simulink model "master_thesis_simulink"  (R2022a)
settings: Solver=VariableStepAuto  StartTime=0.0  StopTime=p_0p.time(end)  FixedStep=0.001  RelTol=1e-3
values from neighbouring files (symbols this model uses):
  markers_forearm = [0.00210510253906 -0.143263397217 -0.00798474121094]    [markers_forearm.mat]
  markers_shoulder = [0.010127746582 -0.151647644043 -0.0119686279297]    [markers_shoulder.mat]
undefined symbols (not defined in the file or in its folder): arm, DiscIntNeverNeededParam, Discrete, ekf, kf, LS, m, markers_hand, n, noise, q0, q0_LS, q0_model, sample_Time, selected, state_observer, Time, tSh_0_0Conf, X, Y, Z
libraries: sm_lib x2029, nesl_utility x1553, robotlib x75, ctrlSharedLib x8
(part 1 of 70)
settings Model: Creator=gioel  LastModifiedBy=gioel
settings DebuggingCC: SignalInfNanChecking=error  InheritedTsInSrcMsg=none

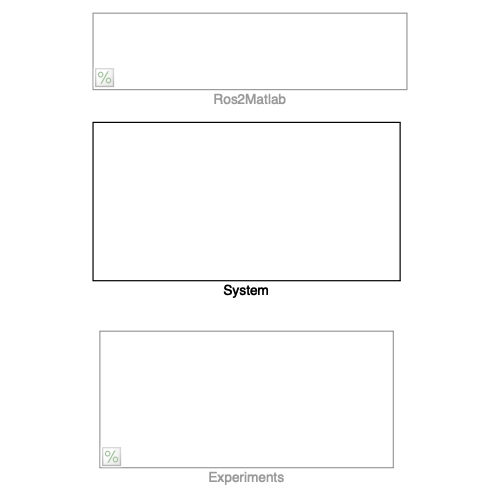
[thumbnail: Simulink's stored preview of the top-level diagram]
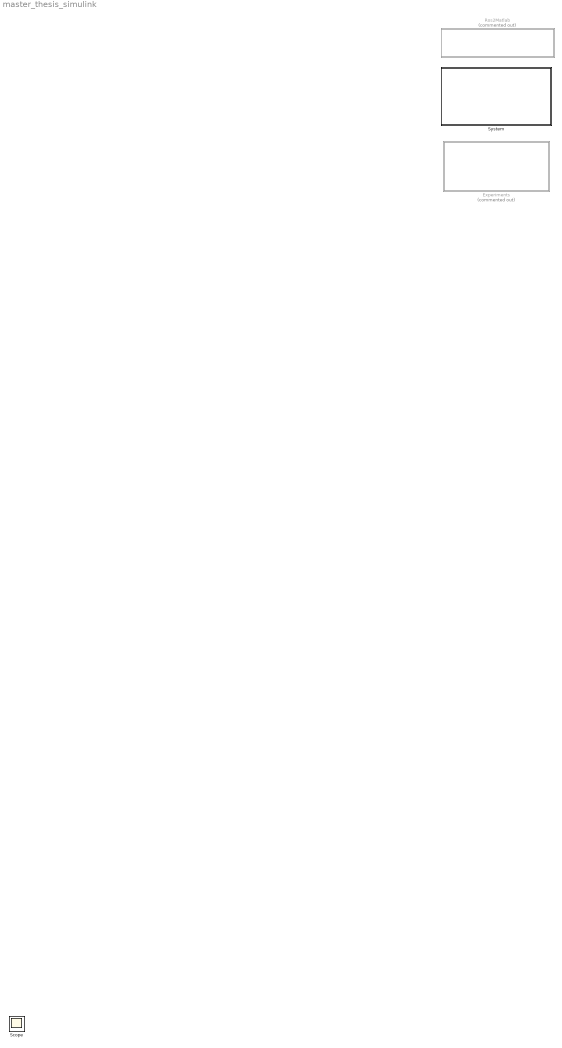
== system master_thesis_simulink ==
  Experiments : Subsystem  Commented=on
  Ros2Matlab : Subsystem  Commented=on
  System : Subsystem
  Scope : Scope

== system master_thesis_simulink/Experiments ==
  S0_F1_H2 : Subsystem  Commented=on
  S0_F2_H2 : Subsystem  Commented=on
  S1_F0_H2 : Subsystem  Commented=on
  S1_F0_H3 : Subsystem  Commented=on
  S1_F1_H2 : Subsystem
  S1_F2_H2 : Subsystem  Commented=on
  S2_F0_H2 : Subsystem  Commented=on

== system master_thesis_simulink/Ros2Matlab ==
  S0_F1_H2 : Subsystem  Commented=on
  S0_F2_H2 : Subsystem  Commented=on
  S1_F0_H2 : Subsystem  Commented=on
  S1_F0_H3 : Subsystem  Commented=on
  S1_F1_H2 : Subsystem
  S1_F2_H2 : Subsystem  Commented=on
  S2_F0_H2 : Subsystem  Commented=on

== system master_thesis_simulink/System ==
  note: q1 = shoulder_x
      | q2 = shoulder_y
      | q3 = shoulder_z
      | q4 = elbow_x
      | q5 = wrist_x
      | q6 = wrist_y
      | q7 = wrist_z
  Constant1 : Constant  Value=markers_shoulder
  Constant2 : Constant  Value=markers_forearm
  Constant3 : Constant  Value=markers_hand
  EKF : Subsystem  Commented=on
  EKF1 : Subsystem  Commented=on
  Human arm : Subsystem  Commented=on
  LKF : Subsystem  Commented=on
  LS : Subsystem  Commented=on
  Mux1 : Mux  Inputs=7
  Mux4 : Mux  Inputs=7
  Noisy p : Subsystem  Commented=on
  Noisy pdot : Subsystem  Commented=on
  Ref : FromWorkspace  Commented=on  VariableName=q_trajectory
  Scope : Scope  NumInputPorts=2
  Scope1 : Scope  NumInputPorts=4
  Show Results : Subsystem
  To Workspace : ToWorkspace  VariableName=q  SaveFormat=Structure With Time  SampleTime=-1
  To Workspace2 : ToWorkspace  VariableName=p  SaveFormat=Structure With Time  SampleTime=-1
  To Workspace4 : ToWorkspace  VariableName=qdot  SaveFormat=Structure With Time  SampleTime=-1
  To Workspace6 : ToWorkspace  VariableName=pdot  SaveFormat=Structure With Time  SampleTime=-1
  ZOH : ZeroOrderHold  SampleTime=sample_Time
  ZOH1 : ZeroOrderHold  SampleTime=sample_Time
  ZOH_q : ZeroOrderHold  SampleTime=sample_Time
  tag scope: markers_f=global, markers_h=global, markers_s=global, p=global, p_true=global, pdot=global, pdot_true=global, q=global, qdot=global
  wires:
  Constant1/1 -> [markers_s]
  [qdot6] -> Mux4/6
  [qdot5] -> Mux4/5
  Constant3/1 -> [markers_h]
  [q6] -> Mux1/6
  Constant2/1 -> [markers_f]
  [qdot2] -> Mux4/2
  [q4] -> Mux1/4
  [q7] -> Mux1/7
  Mux4/1 -> [qdot], To Workspace4/1
  [q2] -> Mux1/2
  [q3] -> Mux1/3
  [q1] -> Mux1/1
  [qdot1] -> Mux4/1
  [q5] -> Mux1/5
  [qdot3] -> Mux4/3
  [qdot7] -> Mux4/7
  [qdot4] -> Mux4/4
  [q] -> Scope1/1  "q"
  ZOH/1 -> EKF1/1(u_noisyk), EKF/1(pdot_k), LKF/1(pdot_k)  "pdot_k"
  Human arm/1(p) -> Scope/1, Noisy p/1(p_true), [p_true]  "p_true"
  Human arm/2(pdot) -> Noisy pdot/1(pdot_true), [pdot_true]  "pdot_true"
  LS/1(q_LS) -> Scope1/2  "q_LS"
  EKF/1(" ") -> Scope1/4  "q_EKF"
  [p] -> ZOH1/1
  ZOH1/1 -> EKF1/2(p_noisyk), EKF/2(p_k), LKF/2(p_k)  "p_k"
  [pdot] -> LS/1(pdot), ZOH/1
  Noisy p/1(p) -> Scope/2, [p], To Workspace2/1  "p"
  Noisy pdot/1(pdot) -> To Workspace6/1, [pdot]  "pdot"
  Ref/1 -> Human arm/1(q ref)
  LKF/1(q_KF) -> Scope1/3
  Mux1/1 -> ZOH_q/1
  ZOH_q/1 -> [q], To Workspace/1  "q_k"

== system master_thesis_simulink/Experiments/S0_F1_H2 ==
  Constant : Constant  Value=selected
  Experiments : Subsystem  TreatAsAtomicUnit=on
  If1 : If
  If2 : If
  If3 : If
  MATLAB Function3 : MATLAB Function  TreatAsAtomicUnit=on
  Model validation : Subsystem  Commented=on  TreatAsAtomicUnit=on
  Noise estimation : Subsystem  Commented=on  TreatAsAtomicUnit=on
  Reshape{1,3..5,7..10} (8 alike) : Reshape  OutputDimensionality=Customize  OutputDimensions=[6,6]
  Scope : Scope
  Selector{,2..4,6..9} (8 alike) : Selector  NumberOfDimensions=2  InputPortWidth=36  IndexOptions=Index vector (dialog),Index vector (dialog)  Indices=1:3,1:3  OutputSizes=1,1
  Terminator1 : Terminator
  Terminator2 : Terminator
  Terminator3 : Terminator
  Vector Concatenate1 : Concatenate  NumInputs=3  Mode=Multidimensional array
  Vector Concatenate2 : Concatenate  NumInputs=3  Mode=Multidimensional array
  tag scope: Rpi_W=global, Rvi_W=global
  wires:
  Selector4/1 -> Vector Concatenate1/3
  Reshape5/1 -> Selector4/1
  Vector Concatenate1/1 -> [Rpi_W]
  Constant/1 -> Experiments/3(Selector)
  If2/1 -> Model validation/Action
  If1/1 -> Experiments/Action
  If3/2 -> Terminator2/1
  Selector3/1 -> Vector Concatenate1/2
  Reshape4/1 -> Selector3/1
  [Rpi_W] -> Noise estimation/2(Rpi_W)
  [isNew] -> MATLAB Function3/1(isNew)
  [Rp3_W] -> Reshape4/1
  If3/1 -> Noise estimation/Action
  Selector/1 -> Noise estimation/1(Rp0_W)
  Reshape1/1 -> Selector/1
  Reshape3/1 -> Selector2/1
  MATLAB Function3/1(y) -> If3/1, If2/1, Scope/1, If1/1
  [v_0p] -> Experiments/2(v_0')
  [Rp0_W] -> Reshape1/1
  If2/2 -> Terminator1/1
  [Rp4_W] -> Reshape5/1
  [Rp2_W] -> Reshape3/1
  If1/2 -> Terminator3/1
  Selector2/1 -> Vector Concatenate1/1
  Selector6/1 -> Vector Concatenate2/1
  [Rv2_W] -> Reshape7/1
  [Rv4_W] -> Reshape9/1
  Reshape7/1 -> Selector6/1
  [Rv3_W] -> Reshape8/1
  Reshape8/1 -> Selector7/1
  Selector7/1 -> Vector Concatenate2/2
  Vector Concatenate2/1 -> [Rvi_W]
  Reshape9/1 -> Selector8/1
  Selector8/1 -> Vector Concatenate2/3
  [Rvi_W] -> Noise estimation/4(Rvi_W)
  [Rv0_W] -> Reshape10/1
  Reshape10/1 -> Selector9/1
  Selector9/1 -> Noise estimation/3(Rv0_W)
  [p_0p] -> Model validation/1(p_0'), Experiments/1(p_0')

== system master_thesis_simulink/Experiments/S0_F2_H2 ==
  Constant : Constant  Value=selected
  Experiments : Subsystem  Commented=on  TreatAsAtomicUnit=on
  If1 : If
  If2 : If
  If3 : If
  MATLAB Function3 : MATLAB Function  TreatAsAtomicUnit=on
  Model validation : Subsystem  TreatAsAtomicUnit=on
  Noise estimation : Subsystem  Commented=on  TreatAsAtomicUnit=on
  Reshape{1..10} (10 alike) : Reshape  OutputDimensionality=Customize  OutputDimensions=[6,6]
  Scope : Scope
  Selector{,1..9} (10 alike) : Selector  NumberOfDimensions=2  InputPortWidth=36  IndexOptions=Index vector (dialog),Index vector (dialog)  Indices=1:3,1:3  OutputSizes=1,1
  Terminator1 : Terminator
  Terminator2 : Terminator
  Terminator3 : Terminator
  Vector Concatenate1 : Concatenate  NumInputs=4  Mode=Multidimensional array
  Vector Concatenate2 : Concatenate  NumInputs=4  Mode=Multidimensional array
  tag scope: Rpi_W=global, Rvi_W=global
  wires:
  [p_0p] -> Experiments/1(p_0'), Model validation/1(p_0')
  Selector9/1 -> Noise estimation/3(Rv0_W)
  Reshape10/1 -> Selector9/1
  [Rv0_W] -> Reshape10/1
  [Rvi_W] -> Noise estimation/4(Rvi_W)
  Selector8/1 -> Vector Concatenate2/4
  Reshape9/1 -> Selector8/1
  Vector Concatenate2/1 -> [Rvi_W]
  [Rv1_W] -> Reshape6/1
  Selector7/1 -> Vector Concatenate2/3
  Reshape8/1 -> Selector7/1
  [Rv3_W] -> Reshape8/1
  Reshape7/1 -> Selector6/1
  Reshape6/1 -> Selector5/1
  [Rv4_W] -> Reshape9/1
  Selector5/1 -> Vector Concatenate2/1
  [Rv2_W] -> Reshape7/1
  Selector6/1 -> Vector Concatenate2/2
  Selector2/1 -> Vector Concatenate1/2
  If1/2 -> Terminator3/1
  [Rp2_W] -> Reshape3/1
  Selector1/1 -> Vector Concatenate1/1
  [Rp4_W] -> Reshape5/1
  If2/2 -> Terminator1/1
  Reshape2/1 -> Selector1/1
  [Rp0_W] -> Reshape1/1
  [v_0p] -> Experiments/2(v_0')
  MATLAB Function3/1(y) -> If1/1, Scope/1, If2/1, If3/1
  Reshape3/1 -> Selector2/1
  Reshape1/1 -> Selector/1
  Selector/1 -> Noise estimation/1(Rp0_W)
  If3/1 -> Noise estimation/Action
  [Rp3_W] -> Reshape4/1
  [isNew] -> MATLAB Function3/1(isNew)
  [Rpi_W] -> Noise estimation/2(Rpi_W)
  Reshape4/1 -> Selector3/1
  Selector3/1 -> Vector Concatenate1/3
  If3/2 -> Terminator2/1
  [Rp1_W] -> Reshape2/1
  If1/1 -> Experiments/Action
  If2/1 -> Model validation/Action
  Constant/1 -> Experiments/3(Selector)
  Vector Concatenate1/1 -> [Rpi_W]
  Reshape5/1 -> Selector4/1
  Selector4/1 -> Vector Concatenate1/4

== system master_thesis_simulink/Experiments/S1_F0_H2 ==
  Constant : Constant  Value=selected
  Experiments : Subsystem  TreatAsAtomicUnit=on
  If1 : If
  If2 : If
  If3 : If
  MATLAB Function3 : MATLAB Function  TreatAsAtomicUnit=on
  Model validation : Subsystem  Commented=on  TreatAsAtomicUnit=on
  Noise estimation : Subsystem  Commented=on  TreatAsAtomicUnit=on
  Reshape{1..2,4..6,8..10} (8 alike) : Reshape  OutputDimensionality=Customize  OutputDimensions=[6,6]
  Scope : Scope
  Selector{,1,3..5,7..9} (8 alike) : Selector  NumberOfDimensions=2  InputPortWidth=36  IndexOptions=Index vector (dialog),Index vector (dialog)  Indices=1:3,1:3  OutputSizes=1,1
  Terminator1 : Terminator
  Terminator2 : Terminator
  Terminator3 : Terminator
  Vector Concatenate1 : Concatenate  NumInputs=3  Mode=Multidimensional array
  Vector Concatenate2 : Concatenate  NumInputs=3  Mode=Multidimensional array
  tag scope: Rpi_W=global, Rvi_W=global
  wires:
  Selector4/1 -> Vector Concatenate1/3
  Reshape5/1 -> Selector4/1
  Vector Concatenate1/1 -> [Rpi_W]
  Constant/1 -> Experiments/3(Selector)
  If2/1 -> Model validation/Action
  If1/1 -> Experiments/Action
  [Rp1_W] -> Reshape2/1
  If3/2 -> Terminator2/1
  Selector3/1 -> Vector Concatenate1/2
  Reshape4/1 -> Selector3/1
  [Rpi_W] -> Noise estimation/2(Rpi_W)
  [isNew] -> MATLAB Function3/1(isNew)
  [Rp3_W] -> Reshape4/1
  If3/1 -> Noise estimation/Action
  Selector/1 -> Noise estimation/1(Rp0_W)
  Reshape1/1 -> Selector/1
  MATLAB Function3/1(y) -> If3/1, If2/1, Scope/1, If1/1
  [v_0p] -> Experiments/2(v_0')
  [Rp0_W] -> Reshape1/1
  Reshape2/1 -> Selector1/1
  If2/2 -> Terminator1/1
  [Rp4_W] -> Reshape5/1
  Selector1/1 -> Vector Concatenate1/1
  If1/2 -> Terminator3/1
  Selector5/1 -> Vector Concatenate2/1
  [Rv4_W] -> Reshape9/1
  Reshape6/1 -> Selector5/1
  [Rv3_W] -> Reshape8/1
  Reshape8/1 -> Selector7/1
  Selector7/1 -> Vector Concatenate2/2
  [Rv1_W] -> Reshape6/1
  Vector Concatenate2/1 -> [Rvi_W]
  Reshape9/1 -> Selector8/1
  Selector8/1 -> Vector Concatenate2/3
  [Rvi_W] -> Noise estimation/4(Rvi_W)
  [Rv0_W] -> Reshape10/1
  Reshape10/1 -> Selector9/1
  Selector9/1 -> Noise estimation/3(Rv0_W)
  [p_0p] -> Model validation/1(p_0'), Experiments/1(p_0')

== system master_thesis_simulink/Experiments/S1_F0_H3 ==
  Constant : Constant  Value=selected
  Experiments : Subsystem  Commented=on  TreatAsAtomicUnit=on
  If1 : If
  If2 : If
  If3 : If
  MATLAB Function3 : MATLAB Function  TreatAsAtomicUnit=on
  Model validation : Subsystem  Commented=on  TreatAsAtomicUnit=on
  Noise estimation : Subsystem  TreatAsAtomicUnit=on
  Reshape{1..10} (10 alike) : Reshape  OutputDimensionality=Customize  OutputDimensions=[6,6]
  Scope : Scope
  Selector{,1..9} (10 alike) : Selector  NumberOfDimensions=2  InputPortWidth=36  IndexOptions=Index vector (dialog),Index vector (dialog)  Indices=1:3,1:3  OutputSizes=1,1
  Terminator1 : Terminator
  Terminator2 : Terminator
  Terminator3 : Terminator
  Vector Concatenate1 : Concatenate  NumInputs=4  Mode=Multidimensional array
  Vector Concatenate2 : Concatenate  NumInputs=4  Mode=Multidimensional array
  tag scope: Rpi_W=global, Rvi_W=global
  wires:
  Selector4/1 -> Vector Concatenate1/4
  Reshape5/1 -> Selector4/1
  Vector Concatenate1/1 -> [Rpi_W]
  Constant/1 -> Experiments/3(Selector)
  If2/1 -> Model validation/Action
  If1/1 -> Experiments/Action
  [Rp1_W] -> Reshape2/1
  If3/2 -> Terminator2/1
  Selector3/1 -> Vector Concatenate1/3
  Reshape4/1 -> Selector3/1
  [Rpi_W] -> Noise estimation/2(Rpi_W)
  [isNew] -> MATLAB Function3/1(isNew)
  [Rp3_W] -> Reshape4/1
  If3/1 -> Noise estimation/Action
  Selector/1 -> Noise estimation/1(Rp0_W)
  Reshape1/1 -> Selector/1
  Reshape3/1 -> Selector2/1
  MATLAB Function3/1(y) -> If3/1, If2/1, Scope/1, If1/1
  [v_0p] -> Experiments/2(v_0')
  [Rp0_W] -> Reshape1/1
  Reshape2/1 -> Selector1/1
  If2/2 -> Terminator1/1
  [Rp4_W] -> Reshape5/1
  Selector1/1 -> Vector Concatenate1/1
  [Rp2_W] -> Reshape3/1
  If1/2 -> Terminator3/1
  Selector2/1 -> Vector Concatenate1/2
  Selector6/1 -> Vector Concatenate2/2
  [Rv2_W] -> Reshape7/1
  Selector5/1 -> Vector Concatenate2/1
  [Rv4_W] -> Reshape9/1
  Reshape6/1 -> Selector5/1
  Reshape7/1 -> Selector6/1
  [Rv3_W] -> Reshape8/1
  Reshape8/1 -> Selector7/1
  Selector7/1 -> Vector Concatenate2/3
  [Rv1_W] -> Reshape6/1
  Vector Concatenate2/1 -> [Rvi_W]
  Reshape9/1 -> Selector8/1
  Selector8/1 -> Vector Concatenate2/4
  [Rvi_W] -> Noise estimation/4(Rvi_W)
  [Rv0_W] -> Reshape10/1
  Reshape10/1 -> Selector9/1
  Selector9/1 -> Noise estimation/3(Rv0_W)
  [p_0p] -> Model validation/1(p_0'), Experiments/1(p_0')

== system master_thesis_simulink/Experiments/S1_F1_H2 ==
  Constant : Constant  Value=selected
  Experiments : Subsystem  TreatAsAtomicUnit=on
  Human arm1 : Subsystem
  If1 : If
  If2 : If
  If3 : If
  MATLAB Function3 : MATLAB Function  TreatAsAtomicUnit=on
  Model validation : Subsystem  Commented=on  TreatAsAtomicUnit=on
  Noise estimation : Subsystem  Commented=on  TreatAsAtomicUnit=on
  Reshape{1..10} (10 alike) : Reshape  OutputDimensionality=Customize  OutputDimensions=[6,6]
  Scope : Scope
  Selector{,1..9} (10 alike) : Selector  NumberOfDimensions=2  InputPortWidth=36  IndexOptions=Index vector (dialog),Index vector (dialog)  Indices=1:3,1:3  OutputSizes=1,1
  Terminator1 : Terminator
  Terminator2 : Terminator
  Terminator3 : Terminator
  Vector Concatenate1 : Concatenate  NumInputs=4  Mode=Multidimensional array
  Vector Concatenate2 : Concatenate  NumInputs=4  Mode=Multidimensional array
  tag scope: Rpi_W=global, Rvi_W=global
  wires:
  Selector4/1 -> Vector Concatenate1/4
  Reshape5/1 -> Selector4/1
  Vector Concatenate1/1 -> [Rpi_W]
  Constant/1 -> Experiments/3(Selector)
  If2/1 -> Model validation/Action
  If1/1 -> Experiments/Action
  [Rp1_W] -> Reshape2/1
  If3/2 -> Terminator2/1
  Selector3/1 -> Vector Concatenate1/3
  Reshape4/1 -> Selector3/1
  [Rpi_W] -> Noise estimation/2(Rpi_W)
  [isNew] -> MATLAB Function3/1(isNew)
  [Rp3_W] -> Reshape4/1
  If3/1 -> Noise estimation/Action
  Selector/1 -> Noise estimation/1(Rp0_W)
  Reshape1/1 -> Selector/1
  Reshape3/1 -> Selector2/1
  MATLAB Function3/1(y) -> If3/1, If2/1, Scope/1, If1/1
  [v_0p] -> Experiments/2(v_0')
  [Rp0_W] -> Reshape1/1
  Reshape2/1 -> Selector1/1
  If2/2 -> Terminator1/1
  [Rp4_W] -> Reshape5/1
  Selector1/1 -> Vector Concatenate1/1
  [Rp2_W] -> Reshape3/1
  If1/2 -> Terminator3/1
  Selector2/1 -> Vector Concatenate1/2
  Selector6/1 -> Vector Concatenate2/2
  [Rv2_W] -> Reshape7/1
  Selector5/1 -> Vector Concatenate2/1
  [Rv4_W] -> Reshape9/1
  Reshape6/1 -> Selector5/1
  Reshape7/1 -> Selector6/1
  [Rv3_W] -> Reshape8/1
  Reshape8/1 -> Selector7/1
  Selector7/1 -> Vector Concatenate2/3
  [Rv1_W] -> Reshape6/1
  Vector Concatenate2/1 -> [Rvi_W]
  Reshape9/1 -> Selector8/1
  Selector8/1 -> Vector Concatenate2/4
  [Rvi_W] -> Noise estimation/4(Rvi_W)
  [Rv0_W] -> Reshape10/1
  Reshape10/1 -> Selector9/1
  Selector9/1 -> Noise estimation/3(Rv0_W)
  [p_0p] -> Model validation/1(p_0'), Experiments/1(p_0')
  Experiments/1(Output) -> Human arm1/1(q_EKF)

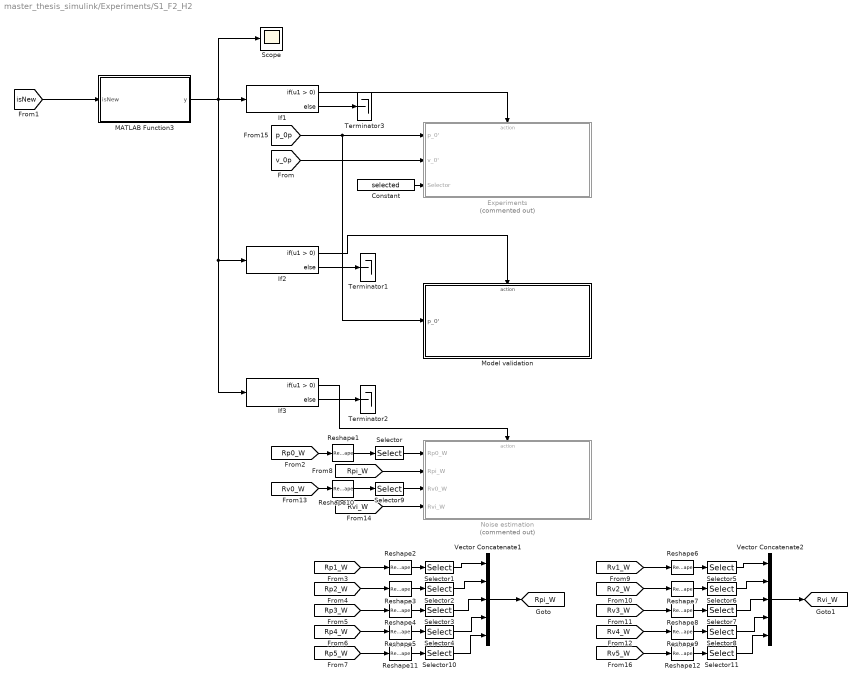
== system master_thesis_simulink/Experiments/S1_F2_H2 ==
  Constant : Constant  Value=selected
  Experiments : Subsystem  Commented=on  TreatAsAtomicUnit=on
  If1 : If
  If2 : If
  If3 : If
  MATLAB Function3 : MATLAB Function  TreatAsAtomicUnit=on
  Model validation : Subsystem  TreatAsAtomicUnit=on
  Noise estimation : Subsystem  Commented=on  TreatAsAtomicUnit=on
  Reshape{1..12} (12 alike) : Reshape  OutputDimensionality=Customize  OutputDimensions=[6,6]
  Scope : Scope
  Selector{,1..11} (12 alike) : Selector  NumberOfDimensions=2  InputPortWidth=36  IndexOptions=Index vector (dialog),Index vector (dialog)  Indices=1:3,1:3  OutputSizes=1,1
  Terminator1 : Terminator
  Terminator2 : Terminator
  Terminator3 : Terminator
  Vector Concatenate1 : Concatenate  NumInputs=5  Mode=Multidimensional array
  Vector Concatenate2 : Concatenate  NumInputs=5  Mode=Multidimensional array
  tag scope: Rpi_W=global, Rvi_W=global
  wires:
  Selector4/1 -> Vector Concatenate1/4
  Reshape5/1 -> Selector4/1
  Vector Concatenate1/1 -> [Rpi_W]
  Constant/1 -> Experiments/3(Selector)
  If2/1 -> Model validation/Action
  If1/1 -> Experiments/Action
  [Rp1_W] -> Reshape2/1
  If3/2 -> Terminator2/1
  Selector3/1 -> Vector Concatenate1/3
  Reshape4/1 -> Selector3/1
  [Rpi_W] -> Noise estimation/2(Rpi_W)
  [isNew] -> MATLAB Function3/1(isNew)
  [Rp3_W] -> Reshape4/1
  If3/1 -> Noise estimation/Action
  Selector/1 -> Noise estimation/1(Rp0_W)
  Reshape1/1 -> Selector/1
  Reshape3/1 -> Selector2/1
  MATLAB Function3/1(y) -> If3/1, If2/1, Scope/1, If1/1
  [v_0p] -> Experiments/2(v_0')
  [Rp0_W] -> Reshape1/1
  Reshape2/1 -> Selector1/1
  If2/2 -> Terminator1/1
  [Rp4_W] -> Reshape5/1
  Selector1/1 -> Vector Concatenate1/1
  [Rp2_W] -> Reshape3/1
  If1/2 -> Terminator3/1
  Selector2/1 -> Vector Concatenate1/2
  Selector6/1 -> Vector Concatenate2/2
  [Rv2_W] -> Reshape7/1
  Selector5/1 -> Vector Concatenate2/1
  [Rv4_W] -> Reshape9/1
  Reshape6/1 -> Selector5/1
  Reshape7/1 -> Selector6/1
  [Rv3_W] -> Reshape8/1
  Reshape8/1 -> Selector7/1
  Selector7/1 -> Vector Concatenate2/3
  [Rv1_W] -> Reshape6/1
  Vector Concatenate2/1 -> [Rvi_W]
  Reshape9/1 -> Selector8/1
  Selector8/1 -> Vector Concatenate2/4
  [Rvi_W] -> Noise estimation/4(Rvi_W)
  [Rv0_W] -> Reshape10/1
  Reshape10/1 -> Selector9/1
  Selector9/1 -> Noise estimation/3(Rv0_W)
  [p_0p] -> Model validation/1(p_0'), Experiments/1(p_0')
  [Rp5_W] -> Reshape11/1
  Reshape11/1 -> Selector10/1
  Selector10/1 -> Vector Concatenate1/5
  Selector11/1 -> Vector Concatenate2/5
  Reshape12/1 -> Selector11/1
  [Rv5_W] -> Reshape12/1

== system master_thesis_simulink/Experiments/S2_F0_H2 ==
  Constant : Constant  Value=selected
  Experiments : Subsystem  TreatAsAtomicUnit=on
  If1 : If
  If2 : If
  If3 : If
  MATLAB Function3 : MATLAB Function  TreatAsAtomicUnit=on
  Model validation : Subsystem  Commented=on  TreatAsAtomicUnit=on
  Noise estimation : Subsystem  Commented=on  TreatAsAtomicUnit=on
  Reshape{1..10} (10 alike) : Reshape  OutputDimensionality=Customize  OutputDimensions=[6,6]
  Scope : Scope
  Selector{,1..9} (10 alike) : Selector  NumberOfDimensions=2  InputPortWidth=36  IndexOptions=Index vector (dialog),Index vector (dialog)  Indices=1:3,1:3  OutputSizes=1,1
  Terminator1 : Terminator
  Terminator2 : Terminator
  Terminator3 : Terminator
  Vector Concatenate1 : Concatenate  NumInputs=4  Mode=Multidimensional array
  Vector Concatenate2 : Concatenate  NumInputs=4  Mode=Multidimensional array
  tag scope: Rpi_W=global, Rvi_W=global
  wires:
  [p_0p] -> Experiments/1(p_0'), Model validation/1(p_0')
  Selector9/1 -> Noise estimation/3(Rv0_W)
  Reshape10/1 -> Selector9/1
  [Rv0_W] -> Reshape10/1
  [Rvi_W] -> Noise estimation/4(Rvi_W)
  Selector8/1 -> Vector Concatenate2/4
  Reshape9/1 -> Selector8/1
  Vector Concatenate2/1 -> [Rvi_W]
  [Rv1_W] -> Reshape6/1
  Selector7/1 -> Vector Concatenate2/3
  Reshape8/1 -> Selector7/1
  [Rv3_W] -> Reshape8/1
  Reshape7/1 -> Selector6/1
  Reshape6/1 -> Selector5/1
  [Rv4_W] -> Reshape9/1
  Selector5/1 -> Vector Concatenate2/1
  [Rv2_W] -> Reshape7/1
  Selector6/1 -> Vector Concatenate2/2
  Selector2/1 -> Vector Concatenate1/2
  If1/2 -> Terminator3/1
  [Rp2_W] -> Reshape3/1
  Selector1/1 -> Vector Concatenate1/1
  [Rp4_W] -> Reshape5/1
  If2/2 -> Terminator1/1
  Reshape2/1 -> Selector1/1
  [Rp0_W] -> Reshape1/1
  [v_0p] -> Experiments/2(v_0')
  MATLAB Function3/1(y) -> If1/1, Scope/1, If2/1, If3/1
  Reshape3/1 -> Selector2/1
  Reshape1/1 -> Selector/1
  Selector/1 -> Noise estimation/1(Rp0_W)
  If3/1 -> Noise estimation/Action
  [Rp3_W] -> Reshape4/1
  [isNew] -> MATLAB Function3/1(isNew)
  [Rpi_W] -> Noise estimation/2(Rpi_W)
  Reshape4/1 -> Selector3/1
  Selector3/1 -> Vector Concatenate1/3
  If3/2 -> Terminator2/1
  [Rp1_W] -> Reshape2/1
  If1/1 -> Experiments/Action
  If2/1 -> Model validation/Action
  Constant/1 -> Experiments/3(Selector)
  Vector Concatenate1/1 -> [Rpi_W]
  Reshape5/1 -> Selector4/1
  Selector4/1 -> Vector Concatenate1/4

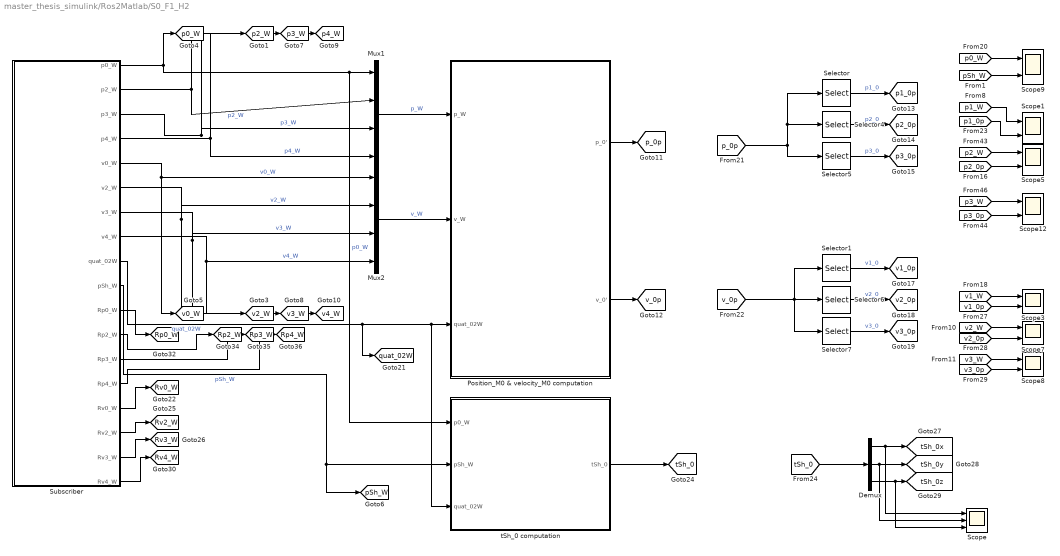
== system master_thesis_simulink/Ros2Matlab/S0_F1_H2 ==
  Demux : Demux  Outputs=3
  Mux1 : Mux
  Mux2 : Mux
  Position_M0 & velocity_M0 computation : Subsystem
  Scope : Scope  NumInputPorts=3
  Scope{1,3,5,7..9,12} (7 alike) : Scope  NumInputPorts=2
  Selector : Selector  InputPortWidth=3*m  IndexOptions=Index vector (dialog)  Indices=1:3  OutputSizes=1
  Selector1 : Selector  InputPortWidth=3*m  IndexOptions=Index vector (dialog)  Indices=1:3  OutputSizes=1
  Selector4 : Selector  InputPortWidth=3*m  IndexOptions=Index vector (dialog)  Indices=4:6  OutputSizes=1
  Selector5 : Selector  InputPortWidth=3*m  IndexOptions=Index vector (dialog)  Indices=7:9  OutputSizes=1
  Selector6 : Selector  InputPortWidth=3*m  IndexOptions=Index vector (dialog)  Indices=4:6  OutputSizes=1
  Selector7 : Selector  InputPortWidth=3*m  IndexOptions=Index vector (dialog)  Indices=7:9  OutputSizes=1
  Subscriber : Subsystem
  tSh_0 computation : Subsystem
  tag scope: Rp0_W=global, Rp2_W=global, Rp3_W=global, Rp4_W=global, Rv0_W=global, Rv2_W=global, Rv3_W=global, Rv4_W=global, p0_W=global, p1_0p=global, p2_0p=global, p2_W=global, p3_0p=global, p3_W=global, p4_W=global, pSh_W=global, p_0p=global, quat_02W=global, tSh_0=global, tSh_0x=global, tSh_0y=global, tSh_0z=global, v0_W=global, v1_0p=global, v2_0p=global, v2_W=global, v3_0p=global, v3_W=global, v4_W=global, v_0p=global
  wires:
  Selector/1 -> [p1_0p]  "p1_0"
  [v1_0p] -> Scope3/2
  Subscriber/14(Rp4_W) -> [Rp4_W]
  Subscriber/12(Rp2_W) -> [Rp2_W]
  [v2_W] -> Scope7/1
  [p3_0p] -> Scope12/2
  tSh_0 computation/1(tSh_0) -> [tSh_0]
  [p1_W] -> Scope1/1
  [v2_0p] -> Scope7/2
  Mux1/1 -> Position_M0 & velocity_M0 computation/1(p_W)  "p_W"
  [p1_0p] -> Scope1/2
  Subscriber/9(quat_02W) -> [quat_02W], tSh_0 computation/3(quat_02W), Position_M0 & velocity_M0 computation/3(quat_02W)  "quat_02W"
  Demux/2 -> Scope/2, [tSh_0y]
  Subscriber/13(Rp3_W) -> [Rp3_W]
  Subscriber/10(pSh_W) -> [pSh_W], tSh_0 computation/2(pSh_W)  "pSh_W"
  Selector1/1 -> [v1_0p]  "v1_0"
  [v3_W] -> Scope8/1
  Demux/1 -> Scope/1, [tSh_0x]
  Subscriber/3(p3_W) -> [p3_W], Mux1/3  "p3_W"
  Subscriber/6(v2_W) -> [v2_W], Mux2/2  "v2_W"
  Subscriber/1(p0_W) -> tSh_0 computation/1(p0_W), Mux1/1, [p0_W]  "p0_W"
  [p2_W] -> Scope5/1
  [p0_W] -> Scope9/1
  Selector6/1 -> [v2_0p]  "v2_0"
  [v1_W] -> Scope3/1
  Subscriber/4(p4_W) -> Mux1/4, [p4_W]  "p4_W"
  [tSh_0] -> Demux/1
  Selector7/1 -> [v3_0p]  "v3_0"
  Subscriber/7(v3_W) -> [v3_W], Mux2/3  "v3_W"
  [p3_W] -> Scope12/1
  [p_0p] -> Selector5/1, Selector/1, Selector4/1
  [p2_0p] -> Scope5/2
  [pSh_W] -> Scope9/2
  Subscriber/8(v4_W) -> [v4_W], Mux2/4  "v4_W"
  [v3_0p] -> Scope8/2
  Subscriber/11(Rp0_W) -> [Rp0_W]
  Selector4/1 -> [p2_0p]  "p2_0"
  Subscriber/2(p2_W) -> Mux1/2, [p2_W]  "p2_W"
  Demux/3 -> Scope/3, [tSh_0z]
  Mux2/1 -> Position_M0 & velocity_M0 computation/2(v_W)  "v_W"
  [v_0p] -> Selector7/1, Selector6/1, Selector1/1
  Selector5/1 -> [p3_0p]  "p3_0"
  Subscriber/5(v0_W) -> [v0_W], Mux2/1  "v0_W"
  Subscriber/15(Rv0_W) -> [Rv0_W]
  Subscriber/16(Rv2_W) -> [Rv2_W]
  Subscriber/17(Rv3_W) -> [Rv3_W]
  Subscriber/18(Rv4_W) -> [Rv4_W]
  Position_M0 & velocity_M0 computation/2(v_0') -> [v_0p]
  Position_M0 & velocity_M0 computation/1(p_0') -> [p_0p]

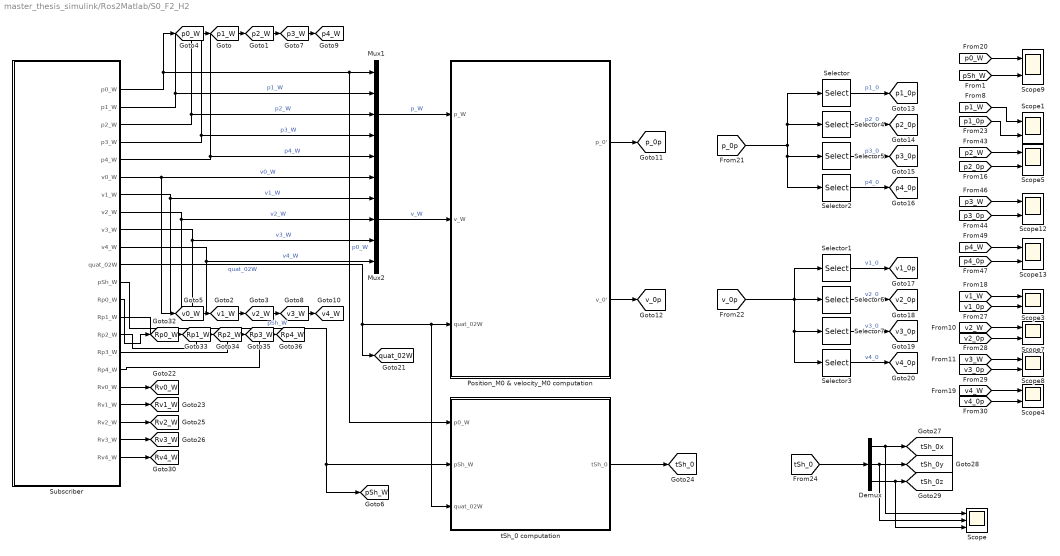
== system master_thesis_simulink/Ros2Matlab/S0_F2_H2 ==
  Demux : Demux  Outputs=3
  Mux1 : Mux  Inputs=5
  Mux2 : Mux  Inputs=5
  Position_M0 & velocity_M0 computation : Subsystem
  Scope : Scope  NumInputPorts=3
  Scope{1,3..5,7..9,12..13} (9 alike) : Scope  NumInputPorts=2
  Selector : Selector  InputPortWidth=3*m  IndexOptions=Index vector (dialog)  Indices=1:3  OutputSizes=1
  Selector1 : Selector  InputPortWidth=3*m  IndexOptions=Index vector (dialog)  Indices=1:3  OutputSizes=1
  Selector2 : Selector  InputPortWidth=3*4  IndexOptions=Index vector (dialog)  Indices=10:12  OutputSizes=1
  Selector3 : Selector  InputPortWidth=3*4  IndexOptions=Index vector (dialog)  Indices=10:12  OutputSizes=1
  Selector4 : Selector  InputPortWidth=3*m  IndexOptions=Index vector (dialog)  Indices=4:6  OutputSizes=1
  Selector5 : Selector  InputPortWidth=3*m  IndexOptions=Index vector (dialog)  Indices=7:9  OutputSizes=1
  Selector6 : Selector  InputPortWidth=3*m  IndexOptions=Index vector (dialog)  Indices=4:6  OutputSizes=1
  Selector7 : Selector  InputPortWidth=3*m  IndexOptions=Index vector (dialog)  Indices=7:9  OutputSizes=1
  Subscriber : Subsystem
  tSh_0 computation : Subsystem
  tag scope: Rp0_W=global, Rp1_W=global, Rp2_W=global, Rp3_W=global, Rp4_W=global, Rv0_W=global, Rv1_W=global, Rv2_W=global, Rv3_W=global, Rv4_W=global, p0_W=global, p1_0p=global, p1_W=global, p2_0p=global, p2_W=global, p3_0p=global, p3_W=global, p4_0p=global, p4_W=global, pSh_W=global, p_0p=global, quat_02W=global, tSh_0=global, tSh_0x=global, tSh_0y=global, tSh_0z=global, v0_W=global, v1_0p=global, v1_W=global, v2_0p=global, v2_W=global, v3_0p=global, v3_W=global, v4_0p=global, v4_W=global, v_0p=global
  wires:
  Selector/1 -> [p1_0p]  "p1_0"
  [p4_W] -> Scope13/1
  [v1_0p] -> Scope3/2
  Subscriber/17(Rp4_W) -> [Rp4_W]
  Subscriber/15(Rp2_W) -> [Rp2_W]
  [v2_W] -> Scope7/1
  [p3_0p] -> Scope12/2
  tSh_0 computation/1(tSh_0) -> [tSh_0]
  [v4_W] -> Scope4/1
  [p1_W] -> Scope1/1
  [v2_0p] -> Scope7/2
  Mux1/1 -> Position_M0 & velocity_M0 computation/1(p_W)  "p_W"
  [p1_0p] -> Scope1/2
  Subscriber/11(quat_02W) -> [quat_02W], tSh_0 computation/3(quat_02W), Position_M0 & velocity_M0 computation/3(quat_02W)  "quat_02W"
  Subscriber/7(v1_W) -> [v1_W], Mux2/2  "v1_W"
  Demux/2 -> Scope/2, [tSh_0y]
  Subscriber/16(Rp3_W) -> [Rp3_W]
  Subscriber/12(pSh_W) -> [pSh_W], tSh_0 computation/2(pSh_W)  "pSh_W"
  Selector1/1 -> [v1_0p]  "v1_0"
  Subscriber/14(Rp1_W) -> [Rp1_W]
  [v3_W] -> Scope8/1
  Demux/1 -> Scope/1, [tSh_0x]
  Subscriber/4(p3_W) -> [p3_W], Mux1/4  "p3_W"
  Subscriber/8(v2_W) -> [v2_W], Mux2/3  "v2_W"
  Subscriber/1(p0_W) -> [p0_W], tSh_0 computation/1(p0_W), Mux1/1  "p0_W"
  [p2_W] -> Scope5/1
  [p0_W] -> Scope9/1
  [p4_0p] -> Scope13/2
  Selector6/1 -> [v2_0p]  "v2_0"
  Selector2/1 -> [p4_0p]  "p4_0"
  [v1_W] -> Scope3/1
  Subscriber/5(p4_W) -> [p4_W], Mux1/5  "p4_W"
  [tSh_0] -> Demux/1
  Selector7/1 -> [v3_0p]  "v3_0"
  Subscriber/9(v3_W) -> [v3_W], Mux2/4  "v3_W"
  [v4_0p] -> Scope4/2
  [p3_W] -> Scope12/1
  [p_0p] -> Selector5/1, Selector2/1, Selector/1, Selector4/1
  [p2_0p] -> Scope5/2
  [pSh_W] -> Scope9/2
  Subscriber/10(v4_W) -> [v4_W], Mux2/5  "v4_W"
  [v3_0p] -> Scope8/2
  Subscriber/13(Rp0_W) -> [Rp0_W]
  Selector4/1 -> [p2_0p]  "p2_0"
  Subscriber/3(p2_W) -> [p2_W], Mux1/3  "p2_W"
  Selector3/1 -> [v4_0p]  "v4_0"
  Demux/3 -> Scope/3, [tSh_0z]
  Mux2/1 -> Position_M0 & velocity_M0 computation/2(v_W)  "v_W"
  Subscriber/2(p1_W) -> [p1_W], Mux1/2  "p1_W"
  [v_0p] -> Selector7/1, Selector3/1, Selector6/1, Selector1/1
  Selector5/1 -> [p3_0p]  "p3_0"
  Subscriber/6(v0_W) -> [v0_W], Mux2/1  "v0_W"
  Subscriber/18(Rv0_W) -> [Rv0_W]
  Subscriber/19(Rv1_W) -> [Rv1_W]
  Subscriber/20(Rv2_W) -> [Rv2_W]
  Subscriber/21(Rv3_W) -> [Rv3_W]
  Subscriber/22(Rv4_W) -> [Rv4_W]
  Position_M0 & velocity_M0 computation/2(v_0') -> [v_0p]
  Position_M0 & velocity_M0 computation/1(p_0') -> [p_0p]

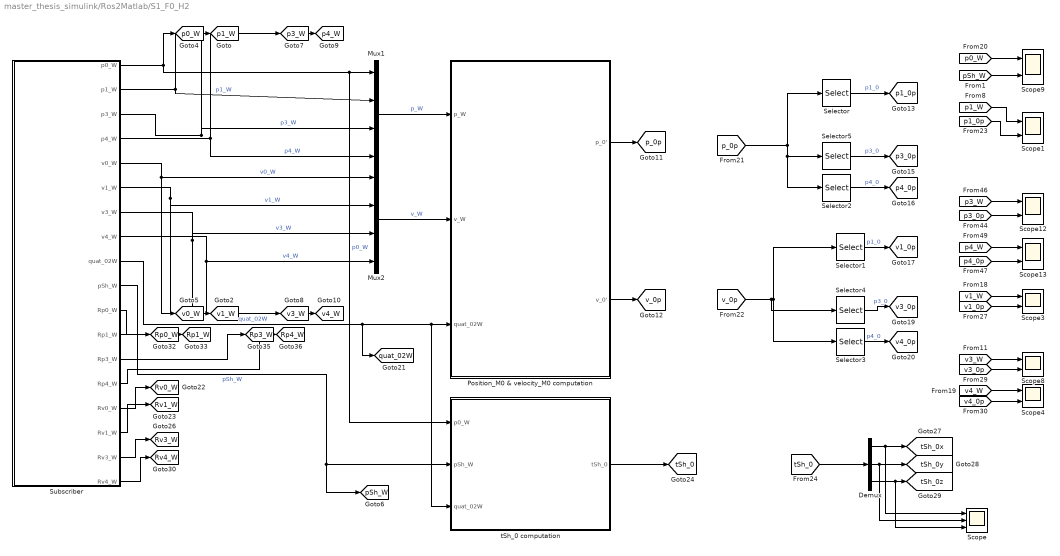
== system master_thesis_simulink/Ros2Matlab/S1_F0_H2 ==
  Demux : Demux  Outputs=3
  Mux1 : Mux
  Mux2 : Mux
  Position_M0 & velocity_M0 computation : Subsystem
  Scope : Scope  NumInputPorts=3
  Scope{1,3..4,8..9,12..13} (7 alike) : Scope  NumInputPorts=2
  Selector : Selector  InputPortWidth=3*m  IndexOptions=Index vector (dialog)  Indices=1:3  OutputSizes=1
  Selector1 : Selector  InputPortWidth=3*m  IndexOptions=Index vector (dialog)  Indices=1:3  OutputSizes=1
  Selector2 : Selector  InputPortWidth=3*3  IndexOptions=Index vector (dialog)  Indices=7:9  OutputSizes=1
  Selector3 : Selector  InputPortWidth=3*3  IndexOptions=Index vector (dialog)  Indices=7:9  OutputSizes=1
  Selector4 : Selector  InputPortWidth=3*m  IndexOptions=Index vector (dialog)  Indices=4:6  OutputSizes=1
  Selector5 : Selector  InputPortWidth=3*m  IndexOptions=Index vector (dialog)  Indices=4:6  OutputSizes=1
  Subscriber : Subsystem
  tSh_0 computation : Subsystem
  tag scope: Rp0_W=global, Rp1_W=global, Rp3_W=global, Rp4_W=global, Rv0_W=global, Rv1_W=global, Rv3_W=global, Rv4_W=global, p0_W=global, p1_0p=global, p1_W=global, p3_0p=global, p3_W=global, p4_0p=global, p4_W=global, pSh_W=global, p_0p=global, quat_02W=global, tSh_0=global, tSh_0x=global, tSh_0y=global, tSh_0z=global, v0_W=global, v1_0p=global, v1_W=global, v3_0p=global, v3_W=global, v4_0p=global, v4_W=global, v_0p=global
  wires:
  Selector/1 -> [p1_0p]  "p1_0"
  [p4_W] -> Scope13/1
  [v1_0p] -> Scope3/2
  Subscriber/14(Rp4_W) -> [Rp4_W]
  [p3_0p] -> Scope12/2
  tSh_0 computation/1(tSh_0) -> [tSh_0]
  [v4_W] -> Scope4/1
  [p1_W] -> Scope1/1
  Mux1/1 -> Position_M0 & velocity_M0 computation/1(p_W)  "p_W"
  [p1_0p] -> Scope1/2
  Subscriber/9(quat_02W) -> [quat_02W], tSh_0 computation/3(quat_02W), Position_M0 & velocity_M0 computation/3(quat_02W)  "quat_02W"
  Subscriber/6(v1_W) -> [v1_W], Mux2/2  "v1_W"
  Demux/2 -> Scope/2, [tSh_0y]
  Subscriber/13(Rp3_W) -> [Rp3_W]
  Subscriber/10(pSh_W) -> [pSh_W], tSh_0 computation/2(pSh_W)  "pSh_W"
  Subscriber/12(Rp1_W) -> [Rp1_W]
  [v3_W] -> Scope8/1
  Demux/1 -> Scope/1, [tSh_0x]
  Subscriber/3(p3_W) -> [p3_W], Mux1/3  "p3_W"
  Subscriber/1(p0_W) -> tSh_0 computation/1(p0_W), Mux1/1, [p0_W]  "p0_W"
  [p0_W] -> Scope9/1
  [p4_0p] -> Scope13/2
  Selector2/1 -> [p4_0p]  "p4_0"
  [v1_W] -> Scope3/1
  Subscriber/4(p4_W) -> Mux1/4, [p4_W]  "p4_W"
  [tSh_0] -> Demux/1
  Subscriber/7(v3_W) -> [v3_W], Mux2/3  "v3_W"
  [v4_0p] -> Scope4/2
  [p3_W] -> Scope12/1
  [p_0p] -> Selector5/1, Selector2/1, Selector/1
  [pSh_W] -> Scope9/2
  Subscriber/8(v4_W) -> [v4_W], Mux2/4  "v4_W"
  [v3_0p] -> Scope8/2
  Subscriber/11(Rp0_W) -> [Rp0_W]
  Demux/3 -> Scope/3, [tSh_0z]
  Mux2/1 -> Position_M0 & velocity_M0 computation/2(v_W)  "v_W"
  Subscriber/2(p1_W) -> Mux1/2, [p1_W]  "p1_W"
  Selector5/1 -> [p3_0p]  "p3_0"
  Subscriber/5(v0_W) -> [v0_W], Mux2/1  "v0_W"
  Subscriber/15(Rv0_W) -> [Rv0_W]
  Subscriber/16(Rv1_W) -> [Rv1_W]
  Subscriber/17(Rv3_W) -> [Rv3_W]
  Subscriber/18(Rv4_W) -> [Rv4_W]
  Position_M0 & velocity_M0 computation/2(v_0') -> [v_0p]
  Position_M0 & velocity_M0 computation/1(p_0') -> [p_0p]
  [v_0p] -> Selector4/1, Selector1/1, Selector3/1
  Selector3/1 -> [v4_0p]  "p4_0"
  Selector4/1 -> [v3_0p]  "p3_0"
  Selector1/1 -> [v1_0p]  "p1_0"

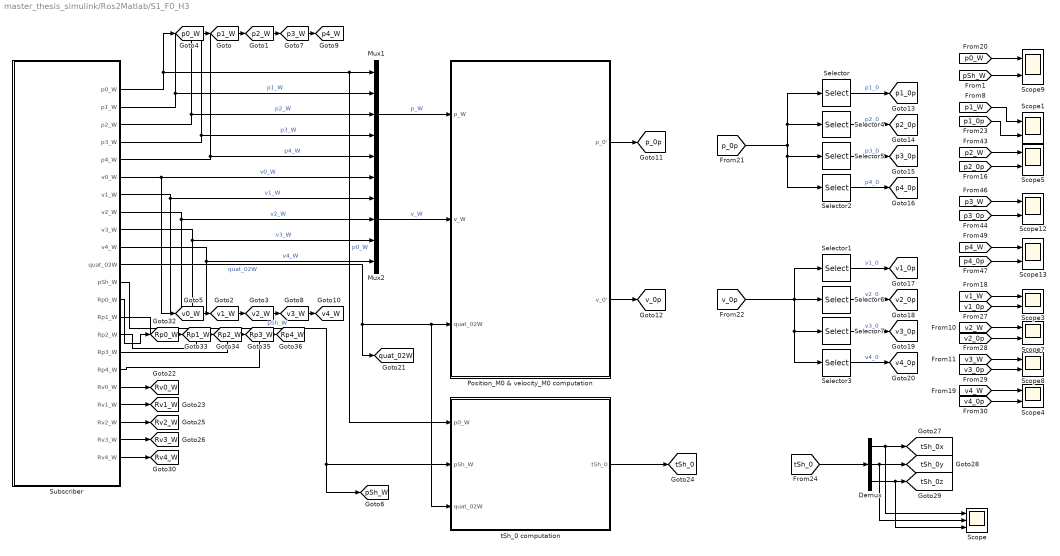
== system master_thesis_simulink/Ros2Matlab/S1_F0_H3 ==
  Demux : Demux  Outputs=3
  Mux1 : Mux  Inputs=5
  Mux2 : Mux  Inputs=5
  Position_M0 & velocity_M0 computation : Subsystem
  Scope : Scope  NumInputPorts=3
  Scope{1,3..5,7..9,12..13} (9 alike) : Scope  NumInputPorts=2
  Selector : Selector  InputPortWidth=3*m  IndexOptions=Index vector (dialog)  Indices=1:3  OutputSizes=1
  Selector1 : Selector  InputPortWidth=3*m  IndexOptions=Index vector (dialog)  Indices=1:3  OutputSizes=1
  Selector2 : Selector  InputPortWidth=3*4  IndexOptions=Index vector (dialog)  Indices=10:12  OutputSizes=1
  Selector3 : Selector  InputPortWidth=3*4  IndexOptions=Index vector (dialog)  Indices=10:12  OutputSizes=1
  Selector4 : Selector  InputPortWidth=3*m  IndexOptions=Index vector (dialog)  Indices=4:6  OutputSizes=1
  Selector5 : Selector  InputPortWidth=3*m  IndexOptions=Index vector (dialog)  Indices=7:9  OutputSizes=1
  Selector6 : Selector  InputPortWidth=3*m  IndexOptions=Index vector (dialog)  Indices=4:6  OutputSizes=1
  Selector7 : Selector  InputPortWidth=3*m  IndexOptions=Index vector (dialog)  Indices=7:9  OutputSizes=1
  Subscriber : Subsystem
  tSh_0 computation : Subsystem
  tag scope: Rp0_W=global, Rp1_W=global, Rp2_W=global, Rp3_W=global, Rp4_W=global, Rv0_W=global, Rv1_W=global, Rv2_W=global, Rv3_W=global, Rv4_W=global, p0_W=global, p1_0p=global, p1_W=global, p2_0p=global, p2_W=global, p3_0p=global, p3_W=global, p4_0p=global, p4_W=global, pSh_W=global, p_0p=global, quat_02W=global, tSh_0=global, tSh_0x=global, tSh_0y=global, tSh_0z=global, v0_W=global, v1_0p=global, v1_W=global, v2_0p=global, v2_W=global, v3_0p=global, v3_W=global, v4_0p=global, v4_W=global, v_0p=global
  wires:
  Selector/1 -> [p1_0p]  "p1_0"
  [p4_W] -> Scope13/1
  [v1_0p] -> Scope3/2
  Subscriber/17(Rp4_W) -> [Rp4_W]
  Subscriber/15(Rp2_W) -> [Rp2_W]
  [v2_W] -> Scope7/1
  [p3_0p] -> Scope12/2
  tSh_0 computation/1(tSh_0) -> [tSh_0]
  [v4_W] -> Scope4/1
  [p1_W] -> Scope1/1
  [v2_0p] -> Scope7/2
  Mux1/1 -> Position_M0 & velocity_M0 computation/1(p_W)  "p_W"
  [p1_0p] -> Scope1/2
  Subscriber/11(quat_02W) -> [quat_02W], tSh_0 computation/3(quat_02W), Position_M0 & velocity_M0 computation/3(quat_02W)  "quat_02W"
  Subscriber/7(v1_W) -> [v1_W], Mux2/2  "v1_W"
  Demux/2 -> Scope/2, [tSh_0y]
  Subscriber/16(Rp3_W) -> [Rp3_W]
  Subscriber/12(pSh_W) -> [pSh_W], tSh_0 computation/2(pSh_W)  "pSh_W"
  Selector1/1 -> [v1_0p]  "v1_0"
  Subscriber/14(Rp1_W) -> [Rp1_W]
  [v3_W] -> Scope8/1
  Demux/1 -> Scope/1, [tSh_0x]
  Subscriber/4(p3_W) -> [p3_W], Mux1/4  "p3_W"
  Subscriber/8(v2_W) -> [v2_W], Mux2/3  "v2_W"
  Subscriber/1(p0_W) -> [p0_W], tSh_0 computation/1(p0_W), Mux1/1  "p0_W"
  [p2_W] -> Scope5/1
  [p0_W] -> Scope9/1
  [p4_0p] -> Scope13/2
  Selector6/1 -> [v2_0p]  "v2_0"
  Selector2/1 -> [p4_0p]  "p4_0"
  [v1_W] -> Scope3/1
  Subscriber/5(p4_W) -> [p4_W], Mux1/5  "p4_W"
  [tSh_0] -> Demux/1
  Selector7/1 -> [v3_0p]  "v3_0"
  Subscriber/9(v3_W) -> [v3_W], Mux2/4  "v3_W"
  [v4_0p] -> Scope4/2
  [p3_W] -> Scope12/1
  [p_0p] -> Selector5/1, Selector2/1, Selector/1, Selector4/1
  [p2_0p] -> Scope5/2
  [pSh_W] -> Scope9/2
  Subscriber/10(v4_W) -> [v4_W], Mux2/5  "v4_W"
  [v3_0p] -> Scope8/2
  Subscriber/13(Rp0_W) -> [Rp0_W]
  Selector4/1 -> [p2_0p]  "p2_0"
  Subscriber/3(p2_W) -> [p2_W], Mux1/3  "p2_W"
  Selector3/1 -> [v4_0p]  "v4_0"
  Demux/3 -> Scope/3, [tSh_0z]
  Mux2/1 -> Position_M0 & velocity_M0 computation/2(v_W)  "v_W"
  Subscriber/2(p1_W) -> [p1_W], Mux1/2  "p1_W"
  [v_0p] -> Selector7/1, Selector3/1, Selector6/1, Selector1/1
  Selector5/1 -> [p3_0p]  "p3_0"
  Subscriber/6(v0_W) -> [v0_W], Mux2/1  "v0_W"
  Subscriber/18(Rv0_W) -> [Rv0_W]
  Subscriber/19(Rv1_W) -> [Rv1_W]
  Subscriber/20(Rv2_W) -> [Rv2_W]
  Subscriber/21(Rv3_W) -> [Rv3_W]
  Subscriber/22(Rv4_W) -> [Rv4_W]
  Position_M0 & velocity_M0 computation/2(v_0') -> [v_0p]
  Position_M0 & velocity_M0 computation/1(p_0') -> [p_0p]

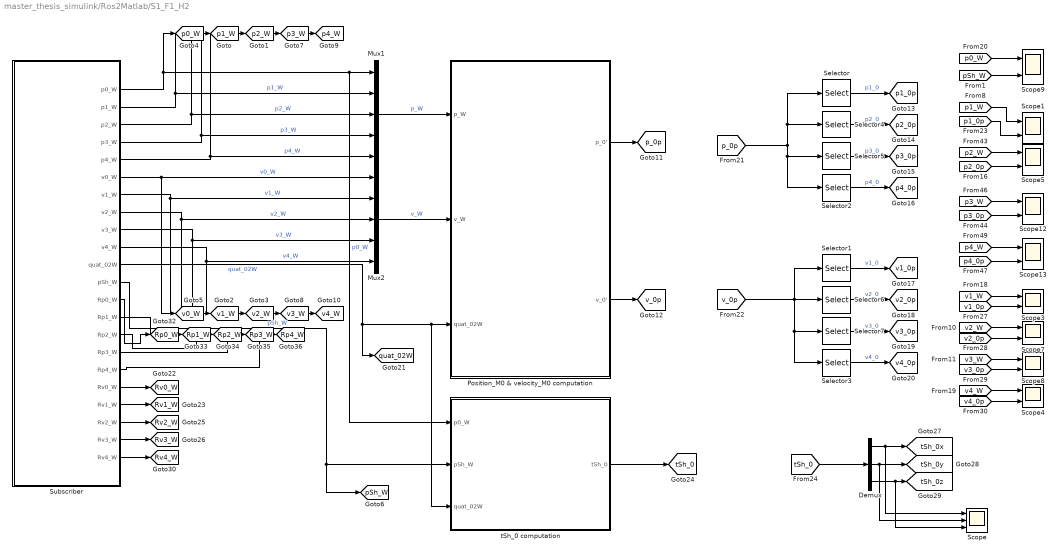
== system master_thesis_simulink/Ros2Matlab/S1_F1_H2 ==
  Demux : Demux  Outputs=3
  Mux1 : Mux  Inputs=5
  Mux2 : Mux  Inputs=5
  Position_M0 & velocity_M0 computation : Subsystem
  Scope : Scope  NumInputPorts=3
  Scope{1,3..5,7..9,12..13} (9 alike) : Scope  NumInputPorts=2
  Selector : Selector  InputPortWidth=3*m  IndexOptions=Index vector (dialog)  Indices=1:3  OutputSizes=1
  Selector1 : Selector  InputPortWidth=3*m  IndexOptions=Index vector (dialog)  Indices=1:3  OutputSizes=1
  Selector2 : Selector  InputPortWidth=3*4  IndexOptions=Index vector (dialog)  Indices=10:12  OutputSizes=1
  Selector3 : Selector  InputPortWidth=3*4  IndexOptions=Index vector (dialog)  Indices=10:12  OutputSizes=1
  Selector4 : Selector  InputPortWidth=3*m  IndexOptions=Index vector (dialog)  Indices=4:6  OutputSizes=1
  Selector5 : Selector  InputPortWidth=3*m  IndexOptions=Index vector (dialog)  Indices=7:9  OutputSizes=1
  Selector6 : Selector  InputPortWidth=3*m  IndexOptions=Index vector (dialog)  Indices=4:6  OutputSizes=1
  Selector7 : Selector  InputPortWidth=3*m  IndexOptions=Index vector (dialog)  Indices=7:9  OutputSizes=1
  Subscriber : Subsystem
  tSh_0 computation : Subsystem
  tag scope: Rp0_W=global, Rp1_W=global, Rp2_W=global, Rp3_W=global, Rp4_W=global, Rv0_W=global, Rv1_W=global, Rv2_W=global, Rv3_W=global, Rv4_W=global, p0_W=global, p1_0p=global, p1_W=global, p2_0p=global, p2_W=global, p3_0p=global, p3_W=global, p4_0p=global, p4_W=global, pSh_W=global, p_0p=global, quat_02W=global, tSh_0=global, tSh_0x=global, tSh_0y=global, tSh_0z=global, v0_W=global, v1_0p=global, v1_W=global, v2_0p=global, v2_W=global, v3_0p=global, v3_W=global, v4_0p=global, v4_W=global, v_0p=global
  wires:
  Selector/1 -> [p1_0p]  "p1_0"
  [p4_W] -> Scope13/1
  [v1_0p] -> Scope3/2
  Subscriber/17(Rp4_W) -> [Rp4_W]
  Subscriber/15(Rp2_W) -> [Rp2_W]
  [v2_W] -> Scope7/1
  [p3_0p] -> Scope12/2
  tSh_0 computation/1(tSh_0) -> [tSh_0]
  [v4_W] -> Scope4/1
  [p1_W] -> Scope1/1
  [v2_0p] -> Scope7/2
  Mux1/1 -> Position_M0 & velocity_M0 computation/1(p_W)  "p_W"
  [p1_0p] -> Scope1/2
  Subscriber/11(quat_02W) -> [quat_02W], tSh_0 computation/3(quat_02W), Position_M0 & velocity_M0 computation/3(quat_02W)  "quat_02W"
  Subscriber/7(v1_W) -> [v1_W], Mux2/2  "v1_W"
  Demux/2 -> Scope/2, [tSh_0y]
  Subscriber/16(Rp3_W) -> [Rp3_W]
  Subscriber/12(pSh_W) -> [pSh_W], tSh_0 computation/2(pSh_W)  "pSh_W"
  Selector1/1 -> [v1_0p]  "v1_0"
  Subscriber/14(Rp1_W) -> [Rp1_W]
  [v3_W] -> Scope8/1
  Demux/1 -> Scope/1, [tSh_0x]
  Subscriber/4(p3_W) -> [p3_W], Mux1/4  "p3_W"
  Subscriber/8(v2_W) -> [v2_W], Mux2/3  "v2_W"
  Subscriber/1(p0_W) -> [p0_W], tSh_0 computation/1(p0_W), Mux1/1  "p0_W"
  [p2_W] -> Scope5/1
  [p0_W] -> Scope9/1
  [p4_0p] -> Scope13/2
  Selector6/1 -> [v2_0p]  "v2_0"
  Selector2/1 -> [p4_0p]  "p4_0"
  [v1_W] -> Scope3/1
  Subscriber/5(p4_W) -> [p4_W], Mux1/5  "p4_W"
  [tSh_0] -> Demux/1
  Selector7/1 -> [v3_0p]  "v3_0"
  Subscriber/9(v3_W) -> [v3_W], Mux2/4  "v3_W"
  [v4_0p] -> Scope4/2
  [p3_W] -> Scope12/1
  [p_0p] -> Selector5/1, Selector2/1, Selector/1, Selector4/1
  [p2_0p] -> Scope5/2
  [pSh_W] -> Scope9/2
  Subscriber/10(v4_W) -> [v4_W], Mux2/5  "v4_W"
  [v3_0p] -> Scope8/2
  Subscriber/13(Rp0_W) -> [Rp0_W]
  Selector4/1 -> [p2_0p]  "p2_0"
  Subscriber/3(p2_W) -> [p2_W], Mux1/3  "p2_W"
  Selector3/1 -> [v4_0p]  "v4_0"
  Demux/3 -> Scope/3, [tSh_0z]
  Mux2/1 -> Position_M0 & velocity_M0 computation/2(v_W)  "v_W"
  Subscriber/2(p1_W) -> [p1_W], Mux1/2  "p1_W"
  [v_0p] -> Selector7/1, Selector3/1, Selector6/1, Selector1/1
  Selector5/1 -> [p3_0p]  "p3_0"
  Subscriber/6(v0_W) -> [v0_W], Mux2/1  "v0_W"
  Subscriber/18(Rv0_W) -> [Rv0_W]
  Subscriber/19(Rv1_W) -> [Rv1_W]
  Subscriber/20(Rv2_W) -> [Rv2_W]
  Subscriber/21(Rv3_W) -> [Rv3_W]
  Subscriber/22(Rv4_W) -> [Rv4_W]
  Position_M0 & velocity_M0 computation/2(v_0') -> [v_0p]
  Position_M0 & velocity_M0 computation/1(p_0') -> [p_0p]

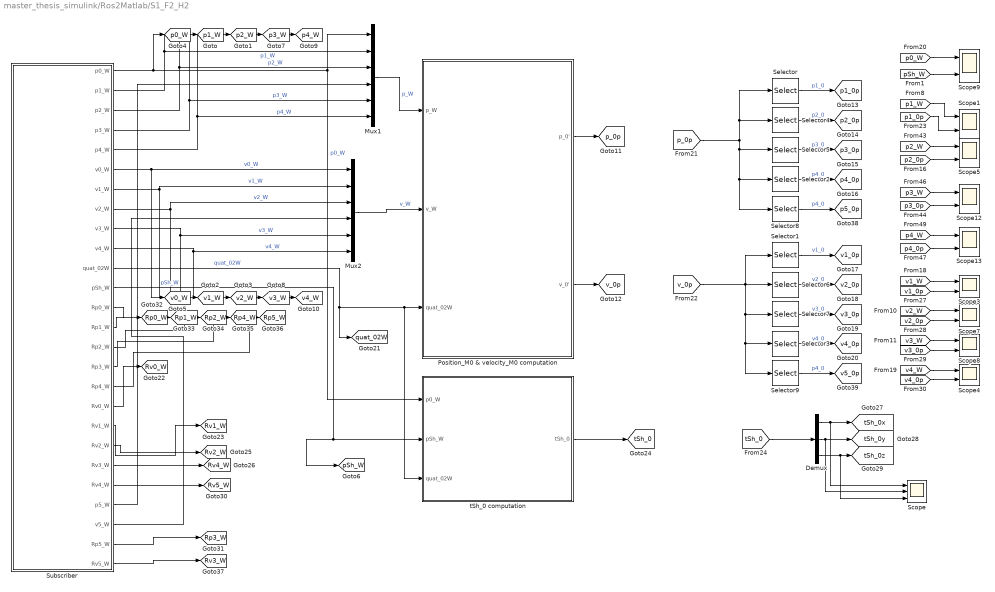
== system master_thesis_simulink/Ros2Matlab/S1_F2_H2 ==
  Demux : Demux  Outputs=3
  Mux1 : Mux  Inputs=6
  Mux2 : Mux  Inputs=6
  Position_M0 & velocity_M0 computation : Subsystem
  Scope : Scope  NumInputPorts=3
  Scope{1,3..5,7..9,12..13} (9 alike) : Scope  NumInputPorts=2
  Selector : Selector  InputPortWidth=15  IndexOptions=Index vector (dialog)  Indices=1:3  OutputSizes=1
  Selector1 : Selector  InputPortWidth=15  IndexOptions=Index vector (dialog)  Indices=1:3  OutputSizes=1
  Selector2 : Selector  InputPortWidth=15  IndexOptions=Index vector (dialog)  Indices=10:12  OutputSizes=1
  Selector3 : Selector  InputPortWidth=15  IndexOptions=Index vector (dialog)  Indices=10:12  OutputSizes=1
  Selector4 : Selector  InputPortWidth=15  IndexOptions=Index vector (dialog)  Indices=4:6  OutputSizes=1
  Selector5 : Selector  InputPortWidth=15  IndexOptions=Index vector (dialog)  Indices=7:9  OutputSizes=1
  Selector6 : Selector  InputPortWidth=15  IndexOptions=Index vector (dialog)  Indices=4:6  OutputSizes=1
  Selector7 : Selector  InputPortWidth=15  IndexOptions=Index vector (dialog)  Indices=7:9  OutputSizes=1
  Selector8 : Selector  InputPortWidth=15  IndexOptions=Index vector (dialog)  Indices=13:15  OutputSizes=1
  Selector9 : Selector  InputPortWidth=15  IndexOptions=Index vector (dialog)  Indices=13:15  OutputSizes=1
  Subscriber : Subsystem
  tSh_0 computation : Subsystem
  tag scope: Rp0_W=global, Rp1_W=global, Rp2_W=global, Rp3_W=global, Rp4_W=global, Rp5_W=global, Rv0_W=global, Rv1_W=global, Rv2_W=global, Rv3_W=global, Rv4_W=global, Rv5_W=global, p0_W=global, p1_0p=global, p1_W=global, p2_0p=global, p2_W=global, p3_0p=global, p3_W=global, p4_0p=global, p4_W=global, p5_0p=global, pSh_W=global, p_0p=global, quat_02W=global, tSh_0=global, tSh_0x=global, tSh_0y=global, tSh_0z=global, v0_W=global, v1_0p=global, v1_W=global, v2_0p=global, v2_W=global, v3_0p=global, v3_W=global, v4_0p=global, v4_W=global, v5_0p=global, v_0p=global
  wires:
  Position_M0 & velocity_M0 computation/1(p_0') -> [p_0p]
  Position_M0 & velocity_M0 computation/2(v_0') -> [v_0p]
  Subscriber/22(Rv4_W) -> [Rv5_W]
  Subscriber/21(Rv3_W) -> [Rv4_W]
  Subscriber/20(Rv2_W) -> [Rv2_W]
  Subscriber/19(Rv1_W) -> [Rv1_W]
  Subscriber/18(Rv0_W) -> [Rv0_W]
  Subscriber/6(v0_W) -> Mux2/1, [v0_W]  "v0_W"
  Selector5/1 -> [p3_0p]  "p3_0"
  [v_0p] -> Selector1/1, Selector6/1, Selector9/1, Selector3/1, Selector7/1
  Subscriber/2(p1_W) -> Mux1/2, [p1_W]  "p1_W"
  Mux2/1 -> Position_M0 & velocity_M0 computation/2(v_W)  "v_W"
  Demux/3 -> [tSh_0z], Scope/3
  Selector3/1 -> [v4_0p]  "v4_0"
  Subscriber/3(p2_W) -> Mux1/3, [p2_W]  "p2_W"
  Selector4/1 -> [p2_0p]  "p2_0"
  Subscriber/13(Rp0_W) -> [Rp0_W]
  [v3_0p] -> Scope8/2
  Subscriber/10(v4_W) -> [v4_W], Mux2/6  "v4_W"
  [pSh_W] -> Scope9/2
  [p2_0p] -> Scope5/2
  [p_0p] -> Selector4/1, Selector/1, Selector8/1, Selector2/1, Selector5/1
  [p3_W] -> Scope12/1
  [v4_0p] -> Scope4/2
  Subscriber/9(v3_W) -> [v3_W], Mux2/5  "v3_W"
  Selector7/1 -> [v3_0p]  "v3_0"
  [tSh_0] -> Demux/1
  Subscriber/5(p4_W) -> Mux1/6, [p4_W]  "p4_W"
  [v1_W] -> Scope3/1
  Selector2/1 -> [p4_0p]  "p4_0"
  Selector6/1 -> [v2_0p]  "v2_0"
  [p4_0p] -> Scope13/2
  [p0_W] -> Scope9/1
  [p2_W] -> Scope5/1
  Subscriber/1(p0_W) -> Mux1/1, tSh_0 computation/1(p0_W), [p0_W]  "p0_W"
  Subscriber/8(v2_W) -> Mux2/3, [v2_W]  "v2_W"
  Subscriber/4(p3_W) -> Mux1/5, [p3_W]  "p3_W"
  Demux/1 -> [tSh_0x], Scope/1
  [v3_W] -> Scope8/1
  Subscriber/14(Rp1_W) -> [Rp1_W]
  Selector1/1 -> [v1_0p]  "v1_0"
  Subscriber/12(pSh_W) -> [pSh_W], tSh_0 computation/2(pSh_W)  "pSh_W"
  Subscriber/16(Rp3_W) -> [Rp4_W]
  Demux/2 -> [tSh_0y], Scope/2
  Subscriber/7(v1_W) -> Mux2/2, [v1_W]  "v1_W"
  Subscriber/11(quat_02W) -> Position_M0 & velocity_M0 computation/3(quat_02W), tSh_0 computation/3(quat_02W), [quat_02W]  "quat_02W"
  [p1_0p] -> Scope1/2
  Mux1/1 -> Position_M0 & velocity_M0 computation/1(p_W)  "p_W"
  [v2_0p] -> Scope7/2
  [p1_W] -> Scope1/1
  [v4_W] -> Scope4/1
  tSh_0 computation/1(tSh_0) -> [tSh_0]
  [p3_0p] -> Scope12/2
  [v2_W] -> Scope7/1
  Subscriber/15(Rp2_W) -> [Rp2_W]
  Subscriber/17(Rp4_W) -> [Rp5_W]
  [v1_0p] -> Scope3/2
  [p4_W] -> Scope13/1
  Selector/1 -> [p1_0p]  "p1_0"
  Subscriber/23(p5_W) -> Mux1/4
  Subscriber/24(v5_W) -> Mux2/4
  Subscriber/25(Rp5_W) -> [Rp3_W]
  Subscriber/26(Rv5_W) -> [Rv3_W]
  Selector8/1 -> [p5_0p]  "p4_0"
  Selector9/1 -> [v5_0p]  "p4_0"

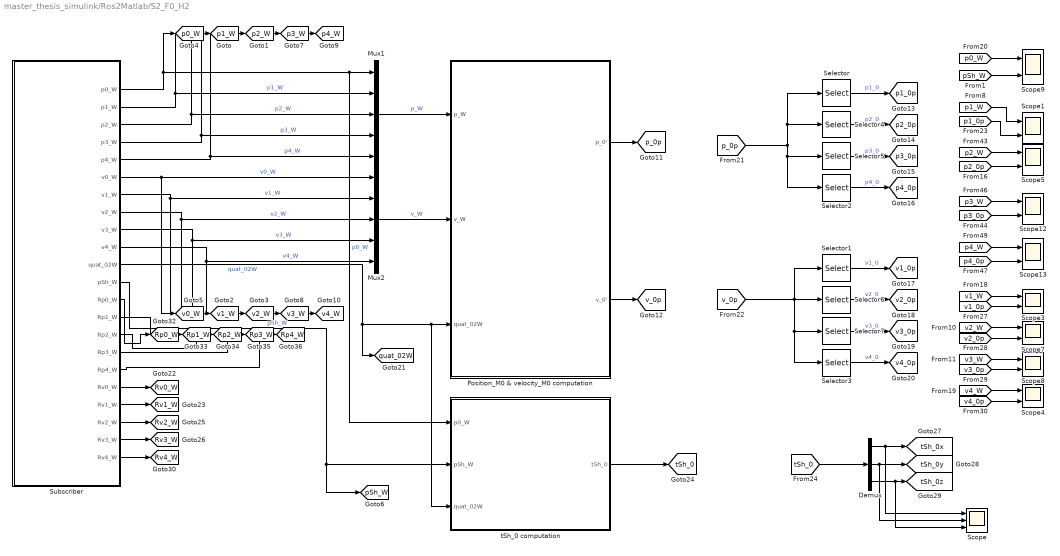
== system master_thesis_simulink/Ros2Matlab/S2_F0_H2 ==
  Demux : Demux  Outputs=3
  Mux1 : Mux  Inputs=5
  Mux2 : Mux  Inputs=5
  Position_M0 & velocity_M0 computation : Subsystem
  Scope : Scope  NumInputPorts=3
  Scope{1,3..5,7..9,12..13} (9 alike) : Scope  NumInputPorts=2
  Selector : Selector  InputPortWidth=3*m  IndexOptions=Index vector (dialog)  Indices=1:3  OutputSizes=1
  Selector1 : Selector  InputPortWidth=3*m  IndexOptions=Index vector (dialog)  Indices=1:3  OutputSizes=1
  Selector2 : Selector  InputPortWidth=3*4  IndexOptions=Index vector (dialog)  Indices=10:12  OutputSizes=1
  Selector3 : Selector  InputPortWidth=3*4  IndexOptions=Index vector (dialog)  Indices=10:12  OutputSizes=1
  Selector4 : Selector  InputPortWidth=3*m  IndexOptions=Index vector (dialog)  Indices=4:6  OutputSizes=1
  Selector5 : Selector  InputPortWidth=3*m  IndexOptions=Index vector (dialog)  Indices=7:9  OutputSizes=1
  Selector6 : Selector  InputPortWidth=3*m  IndexOptions=Index vector (dialog)  Indices=4:6  OutputSizes=1
  Selector7 : Selector  InputPortWidth=3*m  IndexOptions=Index vector (dialog)  Indices=7:9  OutputSizes=1
  Subscriber : Subsystem
  tSh_0 computation : Subsystem
  tag scope: Rp0_W=global, Rp1_W=global, Rp2_W=global, Rp3_W=global, Rp4_W=global, Rv0_W=global, Rv1_W=global, Rv2_W=global, Rv3_W=global, Rv4_W=global, p0_W=global, p1_0p=global, p1_W=global, p2_0p=global, p2_W=global, p3_0p=global, p3_W=global, p4_0p=global, p4_W=global, pSh_W=global, p_0p=global, quat_02W=global, tSh_0=global, tSh_0x=global, tSh_0y=global, tSh_0z=global, v0_W=global, v1_0p=global, v1_W=global, v2_0p=global, v2_W=global, v3_0p=global, v3_W=global, v4_0p=global, v4_W=global, v_0p=global
  wires:
  Selector/1 -> [p1_0p]  "p1_0"
  [p4_W] -> Scope13/1
  [v1_0p] -> Scope3/2
  Subscriber/17(Rp4_W) -> [Rp4_W]
  Subscriber/15(Rp2_W) -> [Rp2_W]
  [v2_W] -> Scope7/1
  [p3_0p] -> Scope12/2
  tSh_0 computation/1(tSh_0) -> [tSh_0]
  [v4_W] -> Scope4/1
  [p1_W] -> Scope1/1
  [v2_0p] -> Scope7/2
  Mux1/1 -> Position_M0 & velocity_M0 computation/1(p_W)  "p_W"
  [p1_0p] -> Scope1/2
  Subscriber/11(quat_02W) -> [quat_02W], tSh_0 computation/3(quat_02W), Position_M0 & velocity_M0 computation/3(quat_02W)  "quat_02W"
  Subscriber/7(v1_W) -> [v1_W], Mux2/2  "v1_W"
  Demux/2 -> Scope/2, [tSh_0y]
  Subscriber/16(Rp3_W) -> [Rp3_W]
  Subscriber/12(pSh_W) -> [pSh_W], tSh_0 computation/2(pSh_W)  "pSh_W"
  Selector1/1 -> [v1_0p]  "v1_0"
  Subscriber/14(Rp1_W) -> [Rp1_W]
  [v3_W] -> Scope8/1
  Demux/1 -> Scope/1, [tSh_0x]
  Subscriber/4(p3_W) -> [p3_W], Mux1/4  "p3_W"
  Subscriber/8(v2_W) -> [v2_W], Mux2/3  "v2_W"
  Subscriber/1(p0_W) -> [p0_W], tSh_0 computation/1(p0_W), Mux1/1  "p0_W"
  [p2_W] -> Scope5/1
  [p0_W] -> Scope9/1
  [p4_0p] -> Scope13/2
  Selector6/1 -> [v2_0p]  "v2_0"
  Selector2/1 -> [p4_0p]  "p4_0"
  [v1_W] -> Scope3/1
  Subscriber/5(p4_W) -> [p4_W], Mux1/5  "p4_W"
  [tSh_0] -> Demux/1
  Selector7/1 -> [v3_0p]  "v3_0"
  Subscriber/9(v3_W) -> [v3_W], Mux2/4  "v3_W"
  [v4_0p] -> Scope4/2
  [p3_W] -> Scope12/1
  [p_0p] -> Selector5/1, Selector2/1, Selector/1, Selector4/1
  [p2_0p] -> Scope5/2
  [pSh_W] -> Scope9/2
  Subscriber/10(v4_W) -> [v4_W], Mux2/5  "v4_W"
  [v3_0p] -> Scope8/2
  Subscriber/13(Rp0_W) -> [Rp0_W]
  Selector4/1 -> [p2_0p]  "p2_0"
  Subscriber/3(p2_W) -> [p2_W], Mux1/3  "p2_W"
  Selector3/1 -> [v4_0p]  "v4_0"
  Demux/3 -> Scope/3, [tSh_0z]
  Mux2/1 -> Position_M0 & velocity_M0 computation/2(v_W)  "v_W"
  Subscriber/2(p1_W) -> [p1_W], Mux1/2  "p1_W"
  [v_0p] -> Selector7/1, Selector3/1, Selector6/1, Selector1/1
  Selector5/1 -> [p3_0p]  "p3_0"
  Subscriber/6(v0_W) -> [v0_W], Mux2/1  "v0_W"
  Subscriber/18(Rv0_W) -> [Rv0_W]
  Subscriber/19(Rv1_W) -> [Rv1_W]
  Subscriber/20(Rv2_W) -> [Rv2_W]
  Subscriber/21(Rv3_W) -> [Rv3_W]
  Subscriber/22(Rv4_W) -> [Rv4_W]
  Position_M0 & velocity_M0 computation/2(v_0') -> [v_0p]
  Position_M0 & velocity_M0 computation/1(p_0') -> [p_0p]

== system master_thesis_simulink/System/EKF ==
  pdot_k : Inport
  p_k : Inport  Port=2
  Clock : Clock
  Extended Kalman Filter : MATLAB Function  TreatAsAtomicUnit=on
  Gain1 : Gain  Gain=180/pi
  Gain2 : Gain  Gain=180/pi
  Saturation : Saturate  UpperLimit=[pi/2; pi/10; 2/3*pi; pi/2; pi/4; pi/10; pi/4]  LowerLimit="[-pi/2; -pi/10; -pi/6; 0; -pi/2;  -pi/2; -pi/4]"
  Scope1 : Scope  NumInputPorts=2
  Terminator : Terminator
  To Workspace8 : ToWorkspace  VariableName=q_EKF  SaveFormat=Structure With Time  SampleTime=-1
  " " : Outport
  wires:
  [markers_s] -> Extended Kalman Filter/3(shoulder_variables)
  p_k/1 -> Extended Kalman Filter/1(p_k)
  [markers_h] -> Extended Kalman Filter/5(hand_variables)
  Gain1/1 -> Scope1/2  "q_EKF [deg]"
  Gain2/1 -> Scope1/1  "q_EKF [deg]"
  [q] -> Gain2/1  "q"
  [markers_f] -> Extended Kalman Filter/4(forearm_variables)
  pdot_k/1 -> Extended Kalman Filter/2(pdot_k)
  Extended Kalman Filter/2(Pk1) -> Terminator/1
  Extended Kalman Filter/1(qk1) -> To Workspace8/1, " "/1, Saturation/1  "ekf"
  Saturation/1 -> Gain1/1
  Clock/1 -> Extended Kalman Filter/6(time)

== system master_thesis_simulink/System/EKF1 ==
  u_noisyk : Inport
  p_noisyk : Inport  Port=2
  Extended Kalman Filter : MATLAB Function  TreatAsAtomicUnit=on
  Scope1 : Scope  NumInputPorts=2
  Terminator : Terminator
  wires:
  [markers_h] -> Extended Kalman Filter/5(hand_variables)
  [q] -> Scope1/1  "q"
  p_noisyk/1 -> Extended Kalman Filter/1(pk)
  Extended Kalman Filter/1(qk) -> Scope1/2  "qekf"
  Extended Kalman Filter/2(Pk) -> Terminator/1
  [markers_s] -> Extended Kalman Filter/3(shoulder_variables)
  [markers_f] -> Extended Kalman Filter/4(forearm_variables)
  u_noisyk/1 -> Extended Kalman Filter/2(uk)
